simulink model "GeneratedOriginalNetwork"  (R2024b)
settings: Solver=FixedStepAuto  StartTime=0.0  StopTime=10.0  RelTol=1e-3
undefined symbols (not defined in the file): netOriginal
libraries: dlsequencelib x2, dlutilitylib x1, dlconvfclib x1, dlinputlayernormlib x1, dlactivationlib x1
settings Model: Creator=bzhuang  LastModifiedBy=bzhuang
settings OptimizationCC: DefaultParameterBehavior=Inlined  EnhancedBackFolding=on  PassReuseOutputArgsAs=Individual arguments  ZeroExternalMemoryAtStartup=off  ZeroInternalMemoryAtStartup=off  OptimizeBlockOrder=speed  DifferentSizesBufferReuse=on  OptimizationCustomize=off  EfficientTunableParamExpr=on
settings DebuggingCC: ParameterTunabilityLossMsg=error
settings SFSimCC: MATLABDynamicMemAlloc=off
settings RTWCC: Description=Embedded Coder  SystemTargetFile=ert.tlc  TemplateMakefile=ert_default_tmf
settings CodeAppCC: ForceParamTrailComments=on  IgnoreCustomStorageClasses=off  OperatorAnnotations=on  SimulinkDataObjDesc=on  SFDataObjDesc=on  InsertBlockDesc=on
settings ERTTargetCC: TargetLangStandard=C99 (ISO)  GenerateSampleERTMain=on  ERTCustomFileTemplate=example_file_process.tlc

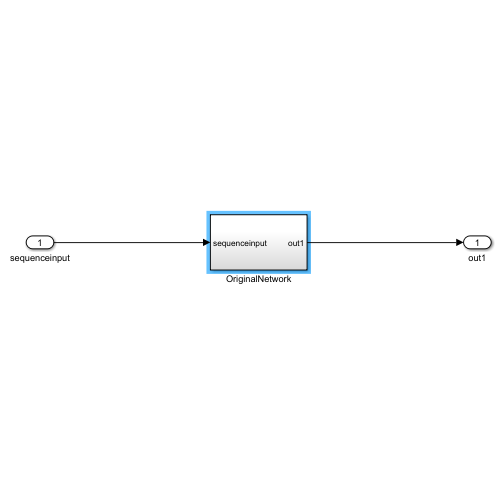
[thumbnail: Simulink's stored preview of the top-level diagram]
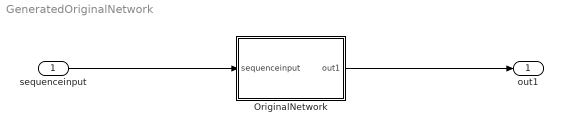
== system GeneratedOriginalNetwork ==
  sequenceinput : Inport  PortDimensions="[10   1]"
  OriginalNetwork : Subsystem
  out1 : Outport
  wires:
  sequenceinput/1 -> OriginalNetwork/1(sequenceinput)
  OriginalNetwork/1(out1) -> out1/1

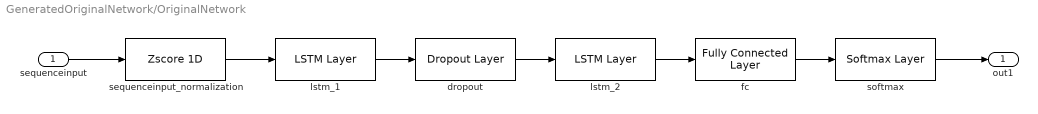
== system GeneratedOriginalNetwork/OriginalNetwork ==
  sequenceinput : Inport  PortDimensions="[10   1]"
  dropout : dlutilitylib/Dropout Layer  SampleTime=-1
  fc : dlconvfclib/Fully Connected Layer  Layer=netOriginal.Layers(5)  OutMin=[]  OutMax=[]  WeightsDataTypeStr=Inherit: Inherit via back propagation  WeightsMin=[]  WeightsMax=[]  BiasDataTypeStr=Inherit: Inherit via back propagation  BiasMin=[]  BiasMax=[]  MatrixMultiplyMin=[]  MatrixMultiplyMax=[]  SampleTime=-1
      settings: DataFormat=C
  lstm_1 : dlsequencelib/LSTM Layer  Layer=netOriginal.Layers(2)  Stateful=on  ApproximationMethod=None  InputWeightsDataTypeStr=Inherit: Inherit via back propagation  InputWeightsMin=[]  InputWeightsMax=[]  RecurrentWeightsDataTypeStr=Inherit: Inherit via back propagation  RecurrentWeightsMin=[]  RecurrentWeightsMax=[]  BiasDataTypeStr=Inherit: Inherit via back propagation  BiasMin=[]  BiasMax=[]  InitialCellStateDataTypeStr=Inherit: Inherit via back propagation  InitialCellStateMin=[]  InitialCellStateMax=[]  CellStateMin=[]  CellStateMax=[]  InitialHiddenStateDataTypeStr=Inherit: Inherit via back propagation  InitialHiddenStateMin=[]  InitialHiddenStateMax=[]  HiddenStateMin=[]  HiddenStateMax=[]  InputWeightsMatrixMultiplyOutMin=[]  InputWeightsMatrixMultiplyOutMax=[]  RecurrentWeightsMatrixMultiplyOutMin=[]  RecurrentWeightsMatrixMultiplyOutMax=[]  LinearGateAddOutMin=[]  LinearGateAddOutMax=[]  CellStateProductOutMin=[]  CellStateProductOutMax=[]  SampleTime=-1
      settings: DataFormat=CT
  lstm_2 : dlsequencelib/LSTM Layer  Layer=netOriginal.Layers(4)  Stateful=on  ApproximationMethod=None  InputWeightsDataTypeStr=Inherit: Inherit via back propagation  InputWeightsMin=[]  InputWeightsMax=[]  RecurrentWeightsDataTypeStr=Inherit: Inherit via back propagation  RecurrentWeightsMin=[]  RecurrentWeightsMax=[]  BiasDataTypeStr=Inherit: Inherit via back propagation  BiasMin=[]  BiasMax=[]  InitialCellStateDataTypeStr=Inherit: Inherit via back propagation  InitialCellStateMin=[]  InitialCellStateMax=[]  CellStateMin=[]  CellStateMax=[]  InitialHiddenStateDataTypeStr=Inherit: Inherit via back propagation  InitialHiddenStateMin=[]  InitialHiddenStateMax=[]  HiddenStateMin=[]  HiddenStateMax=[]  InputWeightsMatrixMultiplyOutMin=[]  InputWeightsMatrixMultiplyOutMax=[]  RecurrentWeightsMatrixMultiplyOutMin=[]  RecurrentWeightsMatrixMultiplyOutMax=[]  LinearGateAddOutMin=[]  LinearGateAddOutMax=[]  CellStateProductOutMin=[]  CellStateProductOutMax=[]  SampleTime=-1
      settings: DataFormat=CT
  sequenceinput_normalization : dlinputlayernormlib/Zscore 1D  Layer=netOriginal.Layers(1)  OutMin=[]  OutMax=[]  MeanDataTypeStr=Inherit: Inherit via back propagation  MeanMin=[]  MeanMax=[]  StandardDeviationDataTypeStr=Inherit: Inherit via back propagation  StandardDeviationMin=[]  StandardDeviationMax=[]  SampleTime=-1
      settings: DataFormat=CT
  softmax : dlactivationlib/Softmax Layer  ApproximationMethod=None  OutMin=[]  OutMax=[]  SampleTime=-1
      settings: DataFormat=C
  out1 : Outport
  wires:
  dropout/1 -> lstm_2/1
  lstm_2/1 -> fc/1
  sequenceinput_normalization/1 -> lstm_1/1
  sequenceinput/1 -> sequenceinput_normalization/1
  lstm_1/1 -> dropout/1
  softmax/1 -> out1/1
  fc/1 -> softmax/1
